simulink model "harmonic_basis"  (R2023a)
settings: Solver=VariableStepAuto  StartTime=0.0  StopTime=10.0  RelTol=1e-3
settings Model: Creator=akb110  LastModifiedBy=akb110

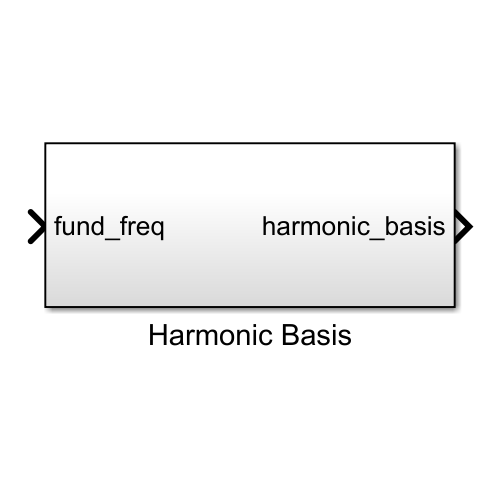
[thumbnail: Simulink's stored preview of the top-level diagram]
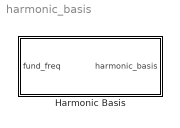
== system harmonic_basis ==
  Harmonic Basis : Subsystem

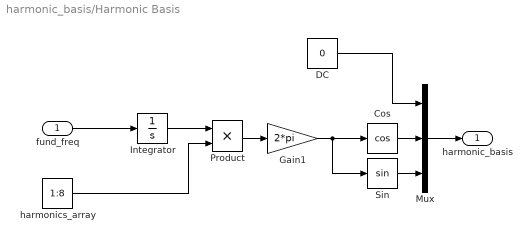
== system harmonic_basis/Harmonic Basis ==
  fund_freq : Inport
  Cos : Trigonometry  Operator=cos
  DC : Constant  Value=0
  Gain1 : Gain  Gain=2*pi
  Integrator : Integrator
  Mux : Mux  Inputs=3
  Product : Product
  Sin : Trigonometry
  harmonics_array : Constant  Value=1:8
  harmonic_basis : Outport  OutDataTypeStr=double  SampleTime=0
  wires:
  Gain1/1 -> Sin/1, Cos/1
  Mux/1 -> harmonic_basis/1
  Integrator/1 -> Product/1
  Cos/1 -> Mux/2
  Product/1 -> Gain1/1
  Sin/1 -> Mux/3
  harmonics_array/1 -> Product/2
  fund_freq/1 -> Integrator/1
  DC/1 -> Mux/1
